simulink model "dmt_sim_alt"  (Simulink 6.0)
settings: Solver=ode45  StartTime=0.0  StopTime=inf  RelTol=1e-3
model workspace: external: M-Code (data not in the file)
undefined symbols (not defined in the file or in its folder): b, slcm
libraries: commdigbbndam2 x20, simulink x3, dspxfrm3 x2, commchan2 x1, commrandsrc2 x1, dspsigattribs x1, dspsrcs4 x1, dspindex x1, commsink2 x1, dspsnks4 x1
CloseFcn:
  | % Clear the signal logging variable
  | clear dmtSigsOut
settings Model: CovMetricSettings=d  Creator=kkwong  LastModifiedBy=fwei  ExtModeAutoUpdateStatusClock=off
settings DataIOCC: SaveOutput=off  SaveTime=off  SignalLoggingName=dmtSigsOut
settings OptimizationCC: BlockReduction=off  BooleanDataType=off
settings DebuggingCC: CheckExecutionContextPreStartOutputMsg=on  CheckExecutionContextRuntimeOutputMsg=on  SolverPrmCheckMsg=none
settings HardwareCC: TargetUnknown=on
settings ModelReferenceCC: UpdateModelReferenceTargets=IfOutOfDate
settings GRTTargetCC: LifeSpan=inf
settings SFSimCC: SFSimApplyToAllLibs=on  SFSimBuildMode=Incremental

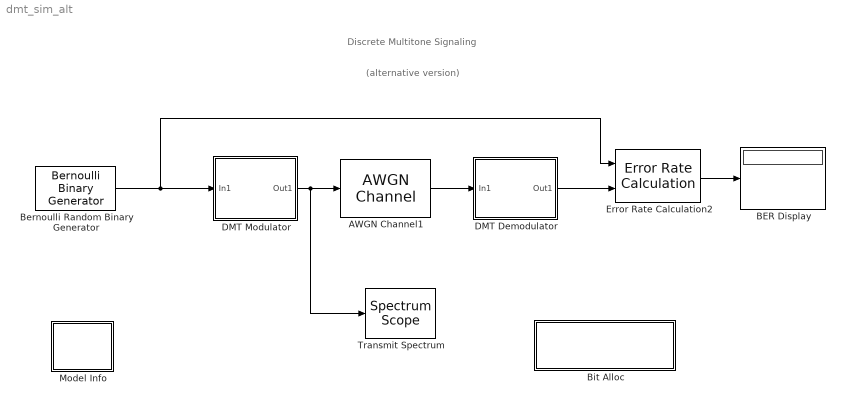
== system dmt_sim_alt ==
  note: Discrete Multitone Signaling
  note: (alternative version)
  AWGN Channel1 : commchan2/AWGN Channel  seed=12345  noiseMode=Variance from mask  EbNodB=10  EsNodB=10  SNRdB=10  bitsPerSym=1  Ps=1  Tsym=1  variance=0.0005
  BER Display : Display
  Bernoulli Random Binary Generator : commrandsrc2/Bernoulli Binary Generator  P=0.5  seed=1  Ts=(1/4000)/sum(b)  frameBased=on  sampPerFrame=sum(b)  orient=off
  Bit Alloc : Subsystem  EnableExecutionContextPropagation=on
      settings: OpenFcn=load('bit_allocation'),plot(b),axis([0 257 1 11]),title('Bit Allocations'),xlabel('Channel'),ylabel('No. Bits')
      mask Display: disp('Load and Plot\nBit Allocation Vector')
  DMT Demodulator : Subsystem  EnableExecutionContextPropagation=on
      mask Display: disp('DMT\nDemodulator')
  DMT Modulator : Subsystem  EnableExecutionContextPropagation=on
      mask Display: disp('DMT\nModulator')
  Error Rate Calculation2 : commsink2/Error Rate Calculation  N=0  st_delay=0  cp_mode=Entire frame  subframe=[]  PMode=Port  WsName=ErrorVec  RsMode2=off  stop=off  numErr=100  maxBits=1000
  Model Info : Subsystem  LoadFcn=slcm LoadBlock;  InitFcn=slcm('UpdateAllCMBlocksInThisModelInit')  EnableExecutionContextPropagation=on  mask(CMBlock){InitialSaveTempField=, InitialBlockCM=none, BlockCM=none, Frame=on, SaveTempField=, DisplayStringWithTags=Info, MaskDisplayString=Info, HorizontalTextAlignment=Center, LeftAlignmentValue=0.5, SourceBlockDiagram=dmt_sim_alt, TagMaxNumber=20, CMTag1=, CMTag2=, CMTag3=, CMTag4=, CMTag5=, CMTag6=, CMTag7=, CMTag8=, CMTag9=, CMTag10=, CMTag11=, CMTag12=, CMTag13=, CMTag14=, CMTag15=, CMTag16=, CMTag17=, CMTag18=, CMTag19=, CMTag20=}
      mask help: This block allows revision control information to be displayed within the model.
      settings: CopyFcn=slcm CopyBlock;  DeleteFcn=slcm Cancel;  PostSaveFcn=slcm('UpdateAllCMBlocksInThisModel')  NameChangeFcn=slcm Rename;  OpenFcn=commdemohelp;
      mask Display: text(str2num(LeftAlignmentValue), 0.5, MaskDisplayString, 'HorizontalAlignment', HorizontalTextAlignment)
  Transmit Spectrum : dspsnks4/Spectrum Scope  ScopeProperties=on  Domain=Frequency  HorizSpan=1  UseBuffer=off  BufferSize=128  Overlap=64  inpFftLenInherit=off  FFTlength=128  numAvg=50  DisplayProperties=off  AxisGrid=on  Memory=off  FrameNumber=on  AxisLegend=off  AxisZoom=off  OpenScopeAtSimStart=on  OpenScopeImmediately=off  FigPos=[13 58 560 460]  AxisProperties=off  XUnits=Hertz  XRange=[0...Fs/2]  InheritXIncr=on  XIncr=1.0  XLabel=Samples  YUnits=dB  YLabel=Magnitude, dB  LineProperties=off
      settings: YMin=-29.4450835994331  YMax=2.87787537591037
  wires:
  Bernoulli Random Binary Generator/1 -> DMT Modulator/1(In1), Error Rate Calculation2/1
  DMT Demodulator/1(Out1) -> Error Rate Calculation2/2
  Error Rate Calculation2/1 -> BER Display/1
  DMT Modulator/1(Out1) -> AWGN Channel1/1, Transmit Spectrum/1
  AWGN Channel1/1 -> DMT Demodulator/1(In1)

== system dmt_sim_alt/Bit Alloc ==

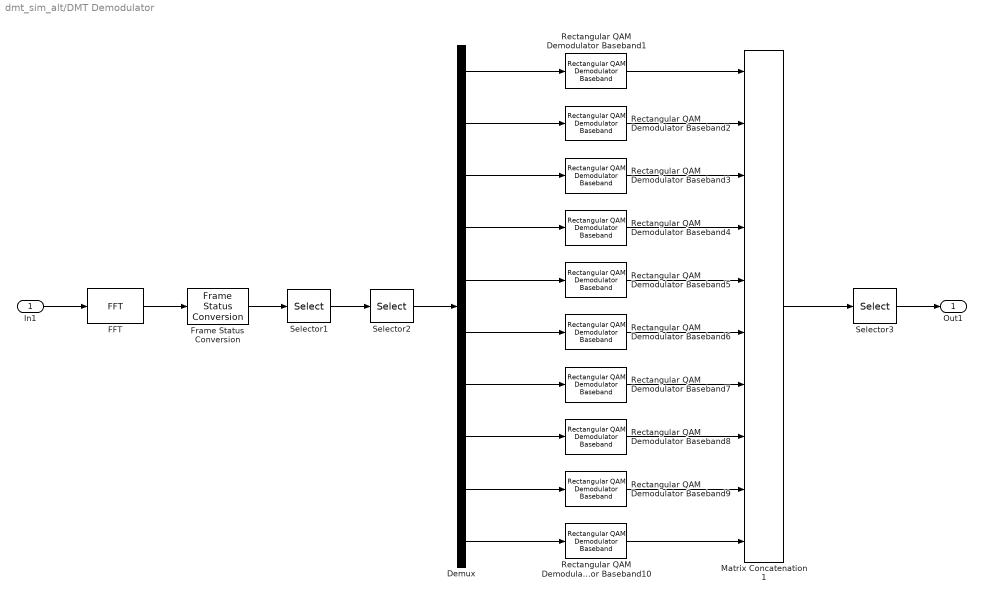
== system dmt_sim_alt/DMT Demodulator ==
  In1 : Inport  LatchInput=off
  Demux : Demux  Outputs=bitalloc(1:end)
  FFT : dspxfrm3/FFT  CompMethod=Table lookup  TableOpt=Speed  BitRevOrder=off  SkipNorm=off  firstCoeffMode=User-defined  firstCoeffWordLength=16  firstCoeffFracLength=15  roundingMode=Floor  overflowMode=off
  Frame Status Conversion : dspsigattribs/Frame Status Conversion  growRefPort=off  outframe=Frame-based
  Matrix Concatenation1 : simulink/Math Operations/Matrix Concatenation  numInports=10  catMethod=Vertical
  Rectangular QAM Demodulator Baseband1 : commdigbbndam2/Rectangular QAM Demodulator Baseband  M=2^1  OutType=Bit  Dec=Binary  PowType=Min. distance between symbols  MinDist=2  AvgPow=1  PeakPow=1  Ph=0  numSamp=1
  Rectangular QAM Demodulator Baseband10 : commdigbbndam2/Rectangular QAM Demodulator Baseband  M=2^10  OutType=Bit  Dec=Binary  PowType=Min. distance between symbols  MinDist=2  AvgPow=1  PeakPow=1  Ph=0  numSamp=1
  Rectangular QAM Demodulator Baseband2 : commdigbbndam2/Rectangular QAM Demodulator Baseband  M=2^2  OutType=Bit  Dec=Binary  PowType=Min. distance between symbols  MinDist=2  AvgPow=1  PeakPow=1  Ph=0  numSamp=1
  Rectangular QAM Demodulator Baseband3 : commdigbbndam2/Rectangular QAM Demodulator Baseband  M=2^3  OutType=Bit  Dec=Binary  PowType=Min. distance between symbols  MinDist=2  AvgPow=1  PeakPow=1  Ph=0  numSamp=1
  Rectangular QAM Demodulator Baseband4 : commdigbbndam2/Rectangular QAM Demodulator Baseband  M=2^4  OutType=Bit  Dec=Binary  PowType=Min. distance between symbols  MinDist=2  AvgPow=1  PeakPow=1  Ph=0  numSamp=1
  Rectangular QAM Demodulator Baseband5 : commdigbbndam2/Rectangular QAM Demodulator Baseband  M=2^5  OutType=Bit  Dec=Binary  PowType=Min. distance between symbols  MinDist=2  AvgPow=1  PeakPow=1  Ph=0  numSamp=1
  Rectangular QAM Demodulator Baseband6 : commdigbbndam2/Rectangular QAM Demodulator Baseband  M=2^6  OutType=Bit  Dec=Binary  PowType=Min. distance between symbols  MinDist=2  AvgPow=1  PeakPow=1  Ph=0  numSamp=1
  Rectangular QAM Demodulator Baseband7 : commdigbbndam2/Rectangular QAM Demodulator Baseband  M=2^7  OutType=Bit  Dec=Binary  PowType=Min. distance between symbols  MinDist=2  AvgPow=1  PeakPow=1  Ph=0  numSamp=1
  Rectangular QAM Demodulator Baseband8 : commdigbbndam2/Rectangular QAM Demodulator Baseband  M=2^8  OutType=Bit  Dec=Binary  PowType=Min. distance between symbols  MinDist=2  AvgPow=1  PeakPow=1  Ph=0  numSamp=1
  Rectangular QAM Demodulator Baseband9 : commdigbbndam2/Rectangular QAM Demodulator Baseband  M=2^9  OutType=Bit  Dec=Binary  PowType=Min. distance between symbols  MinDist=2  AvgPow=1  PeakPow=1  Ph=0  numSamp=1
  Selector1 : Selector  Elements=[1:length(b)]  InputPortWidth=2*length(b)
  Selector2 : Selector  Elements=scrambled  InputPortWidth=length(b)
  Selector3 : Selector  Elements=J  InputPortWidth=sum(b)
  Out1 : Outport
  wires:
  In1/1 -> FFT/1
  FFT/1 -> Frame Status Conversion/1
  Selector2/1 -> Demux/1
  Selector1/1 -> Selector2/1
  Rectangular QAM Demodulator Baseband2/1 -> Matrix Concatenation1/2
  Rectangular QAM Demodulator Baseband3/1 -> Matrix Concatenation1/3
  Rectangular QAM Demodulator Baseband4/1 -> Matrix Concatenation1/4
  Rectangular QAM Demodulator Baseband5/1 -> Matrix Concatenation1/5
  Rectangular QAM Demodulator Baseband6/1 -> Matrix Concatenation1/6
  Rectangular QAM Demodulator Baseband7/1 -> Matrix Concatenation1/7
  Rectangular QAM Demodulator Baseband8/1 -> Matrix Concatenation1/8
  Rectangular QAM Demodulator Baseband9/1 -> Matrix Concatenation1/9
  Rectangular QAM Demodulator Baseband10/1 -> Matrix Concatenation1/10
  Frame Status Conversion/1 -> Selector1/1
  Selector3/1 -> Out1/1
  Demux/10 -> Rectangular QAM Demodulator Baseband10/1
  Demux/9 -> Rectangular QAM Demodulator Baseband9/1
  Demux/8 -> Rectangular QAM Demodulator Baseband8/1
  Demux/7 -> Rectangular QAM Demodulator Baseband7/1
  Demux/6 -> Rectangular QAM Demodulator Baseband6/1
  Demux/5 -> Rectangular QAM Demodulator Baseband5/1
  Demux/4 -> Rectangular QAM Demodulator Baseband4/1
  Demux/3 -> Rectangular QAM Demodulator Baseband3/1
  Demux/2 -> Rectangular QAM Demodulator Baseband2/1
  Demux/1 -> Rectangular QAM Demodulator Baseband1/1
  Rectangular QAM Demodulator Baseband1/1 -> Matrix Concatenation1/1
  Matrix Concatenation1/1 -> Selector3/1

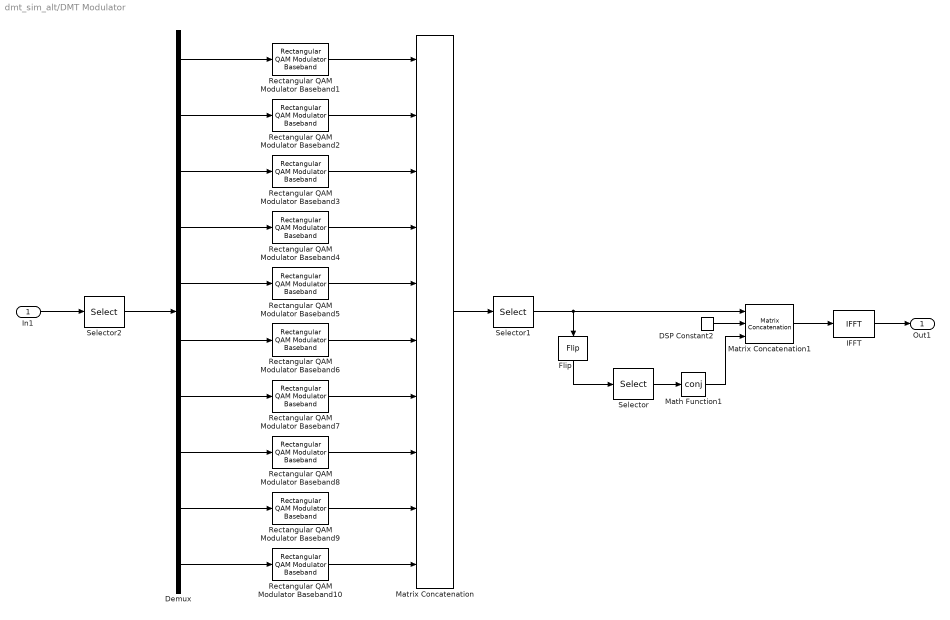
== system dmt_sim_alt/DMT Modulator ==
  In1 : Inport  LatchInput=off
  DSP Constant2 : dspsrcs4/DSP Constant  Value=0  SampleMode=Discrete  discreteOutput=Frame-based  continuousOutput=Sample-based  sampTime=(1/4000)  framePeriod=(1/4000)  dataType=Inherit from 'Constant value'  wordLen=16  udDataType=sfix(16)  fracBitsMode=Best precision  numFracBits=15  InterpretAs1D=off  Ts=(1/4000)  FramebasedOutput=on
  Demux : Demux  Outputs=[[1:10].*bitalloc(1:end)]'
  Flip : dspindex/Flip  Orientation=down  dim=Columns
  IFFT : dspxfrm3/IFFT  CompMethod=Table lookup  TableOpt=Speed  BitRevOrder=off  cs_in=on  SkipNorm=off  mode=Real  firstCoeffMode=User-defined  firstCoeffWordLength=16  firstCoeffFracLength=15  roundingMode=Floor  overflowMode=off
  Math Function1 : Math  Operator=conj  SaturateOnIntegerOverflow=on
  Matrix Concatenation : simulink/Math Operations/Matrix Concatenation  numInports=10  catMethod=Vertical
  Matrix Concatenation1 : simulink/Math Operations/Matrix Concatenation  numInports=3  catMethod=Vertical
  Rectangular QAM Modulator Baseband1 : commdigbbndam2/Rectangular QAM Modulator Baseband  M=2^1  InType=Bit  Enc=Binary  PowType=Min. distance between symbols  MinDist=2  AvgPow=1  PeakPow=1  Ph=0  numSamp=1
  Rectangular QAM Modulator Baseband10 : commdigbbndam2/Rectangular QAM Modulator Baseband  M=2^10  InType=Bit  Enc=Binary  PowType=Min. distance between symbols  MinDist=2  AvgPow=1  PeakPow=1  Ph=0  numSamp=1
  Rectangular QAM Modulator Baseband2 : commdigbbndam2/Rectangular QAM Modulator Baseband  M=2^2  InType=Bit  Enc=Binary  PowType=Min. distance between symbols  MinDist=2  AvgPow=1  PeakPow=1  Ph=0  numSamp=1
  Rectangular QAM Modulator Baseband3 : commdigbbndam2/Rectangular QAM Modulator Baseband  M=2^3  InType=Bit  Enc=Binary  PowType=Min. distance between symbols  MinDist=2  AvgPow=1  PeakPow=1  Ph=0  numSamp=1
  Rectangular QAM Modulator Baseband4 : commdigbbndam2/Rectangular QAM Modulator Baseband  M=2^4  InType=Bit  Enc=Binary  PowType=Min. distance between symbols  MinDist=2  AvgPow=1  PeakPow=1  Ph=0  numSamp=1
  Rectangular QAM Modulator Baseband5 : commdigbbndam2/Rectangular QAM Modulator Baseband  M=2^5  InType=Bit  Enc=Binary  PowType=Min. distance between symbols  MinDist=2  AvgPow=1  PeakPow=1  Ph=0  numSamp=1
  Rectangular QAM Modulator Baseband6 : commdigbbndam2/Rectangular QAM Modulator Baseband  M=2^6  InType=Bit  Enc=Binary  PowType=Min. distance between symbols  MinDist=2  AvgPow=1  PeakPow=1  Ph=0  numSamp=1
  Rectangular QAM Modulator Baseband7 : commdigbbndam2/Rectangular QAM Modulator Baseband  M=2^7  InType=Bit  Enc=Binary  PowType=Min. distance between symbols  MinDist=2  AvgPow=1  PeakPow=1  Ph=0  numSamp=1
  Rectangular QAM Modulator Baseband8 : commdigbbndam2/Rectangular QAM Modulator Baseband  M=2^8  InType=Bit  Enc=Binary  PowType=Min. distance between symbols  MinDist=2  AvgPow=1  PeakPow=1  Ph=0  numSamp=1
  Rectangular QAM Modulator Baseband9 : commdigbbndam2/Rectangular QAM Modulator Baseband  M=2^9  InType=Bit  Enc=Binary  PowType=Min. distance between symbols  MinDist=2  AvgPow=1  PeakPow=1  Ph=0  numSamp=1
  Selector : Selector  Elements=[1:length(b)-1]  InputPortWidth=length(b)
  Selector1 : Selector  Elements=I  InputPortWidth=length(b)
  Selector2 : Selector  Elements=initscram  InputPortWidth=sum(b)
  Out1 : Outport
  wires:
  In1/1 -> Selector2/1
  Matrix Concatenation1/1 -> IFFT/1
  Selector/1 -> Math Function1/1
  Flip/1 -> Selector/1
  IFFT/1 -> Out1/1
  Matrix Concatenation/1 -> Selector1/1
  Selector1/1 -> Flip/1, Matrix Concatenation1/1
  Selector2/1 -> Demux/1
  Math Function1/1 -> Matrix Concatenation1/3
  DSP Constant2/1 -> Matrix Concatenation1/2
  Demux/2 -> Rectangular QAM Modulator Baseband2/1
  Demux/3 -> Rectangular QAM Modulator Baseband3/1
  Demux/4 -> Rectangular QAM Modulator Baseband4/1
  Demux/5 -> Rectangular QAM Modulator Baseband5/1
  Demux/6 -> Rectangular QAM Modulator Baseband6/1
  Demux/7 -> Rectangular QAM Modulator Baseband7/1
  Demux/8 -> Rectangular QAM Modulator Baseband8/1
  Demux/9 -> Rectangular QAM Modulator Baseband9/1
  Demux/10 -> Rectangular QAM Modulator Baseband10/1
  Demux/1 -> Rectangular QAM Modulator Baseband1/1
  Rectangular QAM Modulator Baseband1/1 -> Matrix Concatenation/1
  Rectangular QAM Modulator Baseband2/1 -> Matrix Concatenation/2
  Rectangular QAM Modulator Baseband3/1 -> Matrix Concatenation/3
  Rectangular QAM Modulator Baseband4/1 -> Matrix Concatenation/4
  Rectangular QAM Modulator Baseband5/1 -> Matrix Concatenation/5
  Rectangular QAM Modulator Baseband6/1 -> Matrix Concatenation/6
  Rectangular QAM Modulator Baseband7/1 -> Matrix Concatenation/7
  Rectangular QAM Modulator Baseband8/1 -> Matrix Concatenation/8
  Rectangular QAM Modulator Baseband9/1 -> Matrix Concatenation/9
  Rectangular QAM Modulator Baseband10/1 -> Matrix Concatenation/10

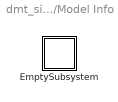
== system dmt_sim_alt/Model Info ==
  EmptySubsystem : Subsystem  EnableExecutionContextPropagation=on

== system dmt_sim_alt/Model Info/EmptySubsystem ==
